simulink model "stabilization"  (R2022b)
settings: Solver=ode14x  StartTime=0.0  StopTime=100  RelTol=1e-3  EnableMultiTasking=on
settings Model: Creator=torre  LastModifiedBy=anver
settings SolverCC: AlgebraicLoopSolver=TrustRegion  AutoInsertRateTranBlk=on
settings DataIOCC: SaveOutput=off  SaveTime=off
settings OptimizationCC: DefaultParameterBehavior=Inlined  InlineInvariantSignals=on  EnhancedBackFolding=on  PassReuseOutputArgsAs=Individual arguments  StateBitsets=on  DataBitsets=on  ZeroExternalMemoryAtStartup=off  ZeroInternalMemoryAtStartup=off  NoFixptDivByZeroProtection=on  LifeSpan=1  OptimizeBlockOrder=speed  DifferentSizesBufferReuse=on  EfficientTunableParamExpr=on
settings DebuggingCC: ParameterTunabilityLossMsg=error  UnconnectedInputMsg=warning  UnconnectedOutputMsg=warning  UnconnectedLineMsg=warning  UnderSpecifiedDimensionMsg=warning
settings HardwareCC: ProdBitPerPointer=32  ProdBitPerSizeT=32  ProdBitPerPtrDiffT=32  ProdLargestAtomicFloat=None  ProdIntDivRoundTo=Floor  ProdWordSize=32  ProdHWDeviceType=Generic->Custom
settings ModelReferenceCC: EnableRefExpFcnMdlSchedulingChecks=on
settings SFSimCC: MATLABDynamicMemAlloc=off
settings RTWCC: Description=Embedded Coder  SystemTargetFile=ert.tlc  TLCOptions=-p0  GenCodeOnly=on  TemplateMakefile=ert_default_tmf  GenerateReport=on  RTWVerbose=off  IncludeHyperlinkInReport=on  LaunchReport=on  DLArmComputeVersion=19.05
settings CodeAppCC: ForceParamTrailComments=on  IgnoreCustomStorageClasses=off  OperatorAnnotations=on  SimulinkDataObjDesc=on  SFDataObjDesc=on  CustomSymbolStrGlobalVar=rt$N$M  CustomSymbolStrType=$N$M  CustomSymbolStrFcn=$N$M$F  CustomSymbolStrMacro=$N$M  InsertBlockDesc=on
settings ERTTargetCC: TargetLangStandard=C99 (ISO)  CodeReplacementLibrary=ISO_C  GenerateSampleERTMain=on  IncludeMdlTerminateFcn=off  SuppressErrorStatus=on  SupportAbsoluteTime=off  PurelyIntegerCode=on  SupportNonFinite=off  SupportComplex=off  InlinedParameterPlacement=NonHierarchical  RootIOFormat=Structure reference  ERTCustomFileTemplate=example_file_process.tlc

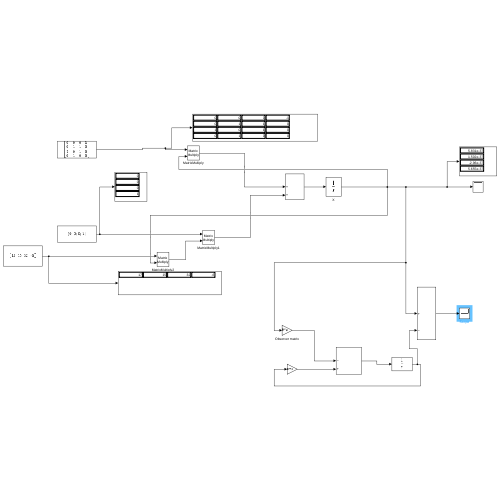
[thumbnail: Simulink's stored preview of the top-level diagram]
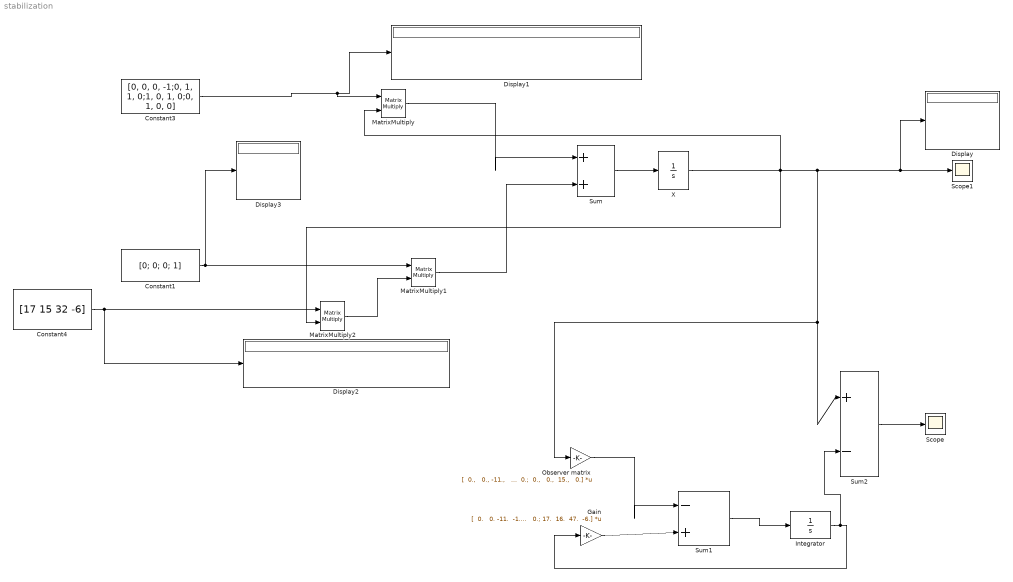
== system stabilization ==
  Constant1 : Constant  Value=[0; 0; 0; 1]  VectorParams1D=off
  Constant3 : Constant  Value=[0, 0, 0, -1;0, 1, 1, 0;1, 0, 1, 0;0, 1, 0, 0]  VectorParams1D=off
  Constant4 : Constant  Value=[17 15 32 -6]  VectorParams1D=off
  Display{,1..3} (4 alike) : Display
  Gain : Gain  Gain="[  0.   0. -11.  -1.;  0.   1.  16.   0.;  1.   0.  -5.   0.; 17.  16.  47.  -6.]"  Multiplication=Matrix(K*u)
  Integrator : Integrator
  MatrixMultiply : Product  Multiplication=Matrix(*)
  MatrixMultiply1 : Product  Multiplication=Matrix(*)
  MatrixMultiply2 : Product  Multiplication=Matrix(*)
  Observer matrix : Gain  Gain="[  0.,   0., -11.,   0.;  0.,   0.,  15.,   0.;  0.,   0.,  -6.,   0.;  0.,   0.,  15.,   0.]"  Multiplication=Matrix(K*u)
  Scope : Scope
  Scope1 : Scope
  Sum : Sum  Inputs=|++
  Sum1 : Sum  Inputs=|-+
  Sum2 : Sum  Inputs=|+-
  X : Integrator  InitialCondition=1
  wires:
  X/1 -> MatrixMultiply2/2, MatrixMultiply/2, Observer matrix/1, Sum2/1, Display/1, Scope1/1
  MatrixMultiply1/1 -> Sum/2
  Sum/1 -> X/1
  MatrixMultiply/1 -> Sum/1
  MatrixMultiply2/1 -> MatrixMultiply1/2
  Constant3/1 -> MatrixMultiply/1, Display1/1
  Constant1/1 -> Display3/1, MatrixMultiply1/1
  Constant4/1 -> Display2/1, MatrixMultiply2/1
  Sum1/1 -> Integrator/1
  Integrator/1 -> Sum2/2, Gain/1
  Gain/1 -> Sum1/2
  Observer matrix/1 -> Sum1/1
  Sum2/1 -> Scope/1
